simulink model "JointSpaceGravityCompensation"  (R2020a)
settings: Solver=VariableStepAuto  StartTime=0.0  StopTime=1.0  RelTol=1e-3
values from neighbouring files (symbols this model uses):
  g = 9.81    [params.m]
  KD = diag([ 20  10  21])    [params.m]
  KP = diag([240 240 200])    [params.m]
libraries: vrlib x1
settings Model: Creator=Sebastiano  LastModifiedBy=Sebastiano

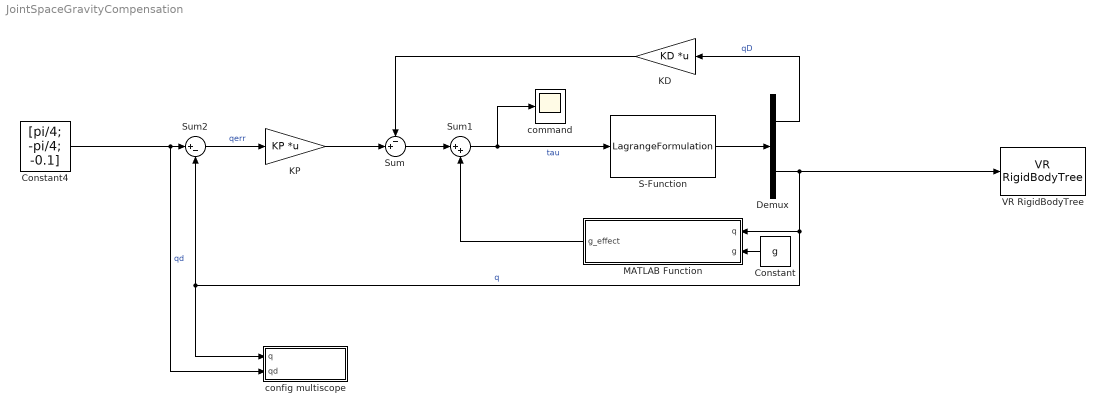
== system JointSpaceGravityCompensation ==
  Constant : Constant  Value=g
  Constant4 : Constant  Value=[pi/4; -pi/4; -0.1]  VectorParams1D=off
  Demux : Demux  Outputs=[3, 3]
  KD : Gain  Gain=KD  Multiplication=Matrix(K*u) (u vector)
  KP : Gain  Gain=KP  Multiplication=Matrix(K*u) (u vector)
  MATLAB Function : MATLAB Function  TreatAsAtomicUnit=on
  S-Function : S-Function  FunctionName=LagrangeFormulation  Parameters=g  SFunctionDeploymentMode=off  EnableBusSupport=off
  Sum : Sum  Inputs=-+|
  Sum1 : Sum  Inputs=|++
  Sum2 : Sum  Inputs=|+-
  VR RigidBodyTree : vrlib/VR RigidBodyTree  RBT=robot  useRBT=on  Ts=-1  ForceViewerOpen=on
      settings: SourceProductBaseCode=SL
  command : Scope
  config multiscope : Subsystem
  wires:
  Demux/2 -> config multiscope/1(q), Sum2/2, MATLAB Function/1(q), VR RigidBodyTree/1  "q"
  Demux/1 -> KD/1  "qD"
  KP/1 -> Sum/2
  Constant4/1 -> config multiscope/2(qd), Sum2/1  "qd"
  Sum2/1 -> KP/1  "qerr"
  MATLAB Function/1(g_effect) -> Sum1/2
  Constant/1 -> MATLAB Function/2(g)
  S-Function/1 -> Demux/1
  Sum1/1 -> S-Function/1, command/1  "tau"
  Sum/1 -> Sum1/1
  KD/1 -> Sum/1

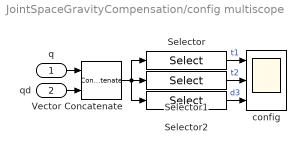
== system JointSpaceGravityCompensation/config multiscope ==
  q : Inport
  qd : Inport  Port=2
  Selector : Selector  NumberOfDimensions=2  InputPortWidth=3  IndexOptions=Index vector (dialog),Select all  Indices=1,7  OutputSizes=6,6
  Selector1 : Selector  NumberOfDimensions=2  InputPortWidth=3  IndexOptions=Index vector (dialog),Select all  Indices=2,7  OutputSizes=6,6
  Selector2 : Selector  NumberOfDimensions=2  InputPortWidth=3  IndexOptions=Index vector (dialog),Select all  Indices=3,7  OutputSizes=6,6
  Vector Concatenate : Concatenate  Mode=Multidimensional array  ConcatenateDimension=2
  config : Scope  NumInputPorts=3
  wires:
  q/1 -> Vector Concatenate/1
  qd/1 -> Vector Concatenate/2
  Selector1/1 -> config/2  "t2"
  Selector/1 -> config/1  "t1"
  Vector Concatenate/1 -> Selector/1, Selector2/1, Selector1/1
  Selector2/1 -> config/3  "d3"

== matlab function JointSpaceGravityCompensation/MATLAB Function ==
  data: q input; g_effect output; g input
function g_effect = gravity(q, g)

g_effect = G_Lagrangian(q, g);
